simulink model "simulink_buck_converter_simpli"  (R2020b)
settings: Solver=ode23tb  StartTime=0  StopTime=t_end_sim  MaxStep=T_s/500  RelTol=1e-3
values from neighbouring files (symbols this model uses):
  C = 10e-6    (= 1e-05)    [Buck.m]    (also in ex6.m)
  D = 0.25    [Buck.m]    (also in ex6.m)
  L = 75e-6    (= 7.5e-05)    [Buck.m]    (also in ex6.m)
  R = 40    [Buck.m]    (also in ex6.m = i)
  V_i = 12    [Buck.m]    (also in ex6.m)
libraries: powerlib x9, powerlib_meascontrol x1
settings Model: Creator=arnaudsaison  LastModifiedBy=arnaudsaison
settings DataIOCC: SaveTime=off  ReturnWorkspaceOutputs=off
settings DebuggingCC: UnconnectedOutputMsg=none
settings HardwareCC: ProdBitPerLong=64  ProdHWDeviceType=Intel->x86-64 (Mac OS X)

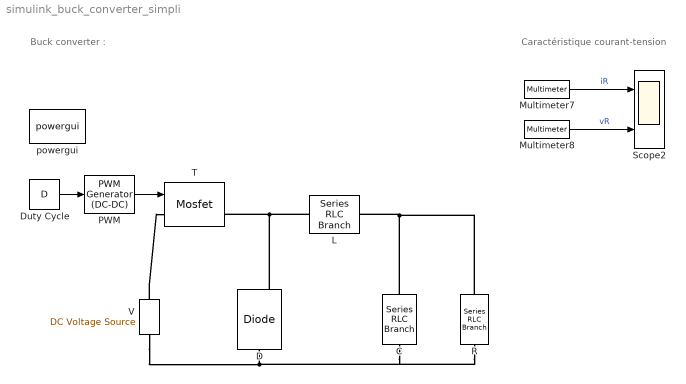
== system simulink_buck_converter_simpli ==
  note: Buck converter :
  note: Caractéristique courant-tension
  C : powerlib/Elements/Series RLC Branch  LConnTagsString=__new0  RConnTagsString=__new0  BranchType=C  Resistance=1  Inductance=1e-3  SetiL0=off  InitialCurrent=0  Capacitance=C  Setx0=off  InitialVoltage=0  Measurements=Branch current
  D : powerlib/Power Electronics/Diode  Ron=0.001 * 0  Lon=0  Vf=0.8 * 0  IC=0  UseSnubber=0  Rs=500  Cs=250e-9  Measurements=on
  Duty Cycle : Constant  Value=D
  L : powerlib/Elements/Series RLC Branch  LConnTagsString=__new0  RConnTagsString=__new0  BranchType=L  Resistance=1  Inductance=L  SetiL0=off  InitialCurrent=0  Capacitance=1e-6  Setx0=off  InitialVoltage=0  Measurements=Branch current
  Multimeter7 : powerlib/Measurements/Multimeter  PhasorSimulation=off  OutputType=Complex  sel=4  L=4  Gain=1  yselected={'Ib: R'};  PSBOutputType=1  PSBequivalent=0  AxesSetting=[0,0.1,-100,100]  Display=0  SavedBlockNames=-11
  Multimeter8 : powerlib/Measurements/Multimeter  PhasorSimulation=off  OutputType=Complex  sel=1  L=4  Gain=1  yselected={'Ub: R'};  PSBOutputType=1  PSBequivalent=0  AxesSetting=[0,0.1,-100,100]  Display=0  SavedBlockNames=-11
  PWM : powerlib_meascontrol/Pulse & Signal Generators/PWM Generator (DC-DC)  Fsw=f_s  Ts=0
  R : powerlib/Elements/Series RLC Branch  LConnTagsString=__new0  RConnTagsString=__new0  BranchType=R  Resistance=R  Inductance=1e-3  SetiL0=off  InitialCurrent=0  Capacitance=1e-6  Setx0=off  InitialVoltage=0  Measurements=Branch voltage and current
  Scope2 : Scope  NumInputPorts=2
  T : powerlib/Power Electronics/Mosfet  Ron=0.1*0  Lon=0  Rd=0.01*0  Vfd=0  IC=0  Rs=1e5  Cs=inf  Measurements=on
  V : powerlib/Electrical Sources/DC Voltage Source  Amplitude=V_i  Measurements=None
  powergui : powerlib/powergui  Priority=1  SimulationMode=Continuous  SampleTime=50e-6  frequency=60  Iterations=50  frequencyindice=0  Pbase=100e6  ErrMax=1e-4  UnitsV=kV  UnitsW=MW  buscounter=0  FunctionMessages=off  echomessages=off  EnableUseOfTLC=off  CurrentSourceSwitches=off  DisableSnubberDevices=off  DisableRonSwitches=off  DisableVfSwitches=off  DisplayEquations=off  AutomaticDiscreteSolvers=off  SolverType=Tustin/Backward Euler (TBE)  Interpol=off  ExternalGateDelay=off  methode=off  Ts=100  x0status=blocks  SPID=on  SwTol=0  HookPort=off  NonlinearTolerance=1e-4  nMaxIteration=100  ContinueOnMaxIteration=off  RestoreLinks=warning  ResistiveCurrentMeasurement=off  Frange=[0:2:500]  Ylog=off  Xlog=on  ShowGrid=off  save=off  variable=ZData  structure=vi3  ZoomFFT=off  StartTime=0.18  cycles=1  DisplayStyle=4  fundamental=50  FreqAxis=on  MaxFrequency=2500  frequencyindicesteady=1  RmsSteady=1  display=off
  wires:
  Duty Cycle/1 -> PWM/1
  PWM/1 -> T/1
  Multimeter7/1 -> Scope2/1  "iR"
  Multimeter8/1 -> Scope2/2  "vR"
  connections:
  V/RConn1 -- T/LConn1
  L/LConn1 -- D/RConn1 -- T/RConn1
  C/LConn1 -- R/LConn1 -- L/RConn1
  V/LConn1 -- R/RConn1 -- C/RConn1 -- D/LConn1
